simulink model "ekviv_prenos_nelin"  (R2018a)
settings: Solver=VariableStepAuto  StartTime=0.0  StopTime=10.0  RelTol=1e-3
settings Model: Creator=vejvarm  LastModifiedBy=vejvarm

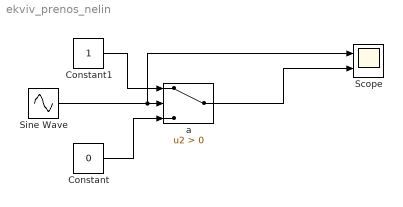
== system ekviv_prenos_nelin ==
  Constant : Constant  Value=0
  Constant1 : Constant
  Scope : Scope  NumInputPorts=2
  Sine Wave : Sin  Amplitude=2  Frequency=2  SampleTime=0
  a : Switch  Criteria=u2 > Threshold
  wires:
  Sine Wave/1 -> Scope/1, a/2
  Constant1/1 -> a/1
  Constant/1 -> a/3
  a/1 -> Scope/2
